simulink model "DC_DC_source_based_matrix_switches1"  (R2023b)
settings: Solver=FixedStepAuto  StartTime=0.0  StopTime=10000  FixedStep=0.01  RelTol=1e-3
InitFcn:
  | %run('D:\Thesis\main.m')
  | %run('E:\Thesis\main.m')
values from neighbouring files (symbols this model uses):
  cell_cap_Ah = 2.2    [find_maximum_ovlp.m]    (also in main.m)
  dst_q_cls = zeros(50, 2)    [main.m]
  dst_trg_soc_av = zeros(50, 1)    [main.m]
  soc = soc_in    [balance_costF.m]    (also in find_maximum_ovlp.m = fix(rand (1, cell_count) * 100); log_clustering.m; main.m = [16   16  50  27  27  23  22  73  73]; plot_final.m)
  src_q_cls = zeros(50, 2)    [main.m]
  src_trg_soc_av = zeros(50, 1)    [main.m]
undefined symbols (not defined in the file or in its folder): Ion, Lithium
libraries: spsIdealSwitchLib x18, spsBatteryLib x10, spsControlledCurrentSourceLib x4, spsVoltageMeasurementLib x4, simulink x2, slpidlib x1, spspowerguiLib x1
(part 2 of 2)

== matlab function DC_DC_source_based_matrix_switches1/DC-DC converter3/MATLAB Function ==
  data: enable input; current_left output; direction input; voltage_left input; voltage_right input; current_right output; current_desired input
function [current_left, current_right] = current_controller(enable, direction, voltage_left, voltage_right, current_desired)    
    current_left = 0;
    current_right = 0;
if(enable)
    %% left side sink, right side source
    if(direction == 0) 
        % variables definition
        current_source = -1 * current_desired;
        voltage_sink = voltage_left;
        voltage_source = voltage_right;

        % input and output power must match
        power_source = current_source * voltage_source;
        power_sink = power_source;
        if(voltage_sink  ~= 0)
            current_sink =  -1 * (power_sink / voltage_sink);
        else
            current_sink = -1 * current_source;
        end
        % power delivery
        if(current_sink > 0)
            current_sink = current_sink * -1;
        end
        if(current_source < 0)
            current_source = current_source * -1;
        end
        current_left = current_sink;
        current_right = current_source;
    %% left side source, right side sink
    elseif(direction == 1)
        % variables definition
        current_source = 1 * current_desired;
        voltage_sink = voltage_right;
        voltage_source = voltage_left;

        % input and output power must match
        power_source = current_source * voltage_source;
        power_sink = power_source;
        if(voltage_sink  ~= 0)
            current_sink =  -1 * (power_sink / voltage_sink);
        else
            current_sink = -1 * current_source;
        end

        % power delivery
        current_left = current_source;
        current_right = current_sink;
    end

else
    current_left = 0;
    current_right = 0;
end
end

== matlab function DC_DC_source_based_matrix_switches1/mcu/demux n ==
  data: u input; s1 output boolean; s2 output boolean; s3 output boolean; s4 output boolean; s5 output boolean; s6 output boolean; s7 output boolean; s8 output boolean; s9 output boolean
function [s1, s2, s3, s4, s5, s6, s7, s8, s9] = demux(u)

    switch(u)
        case 1
            s1 = true; s2 = false; s3 = false; s4 = false; s5 = false; s6 = false; s7 = false; s8 = false; s9 = false;
        case 2      	
            s1 = false; s2 = true; s3 = false; s4 = false; s5 = false; s6 = false; s7 = false; s8 = false; s9 = false;
        case 3      	
            s1 = false; s2 = false; s3 = true; s4 = false; s5 = false; s6 = false; s7 = false; s8 = false; s9 = false;
        case 4      	
            s1 = false; s2 = false; s3 = false; s4 = true; s5 = false; s6 = false; s7 = false; s8 = false; s9 = false;
        case 5      	
            s1 = false; s2 = false; s3 = false; s4 = false; s5 = true; s6 = false; s7 = false; s8 = false; s9 = false;
        case 6      	
            s1 = false; s2 = false; s3 = false; s4 = false; s5 = false; s6 = true; s7 = false; s8 = false; s9 = false;
        case 7      
            s1 = false; s2 = false; s3 = false; s4 = false; s5 = false; s6 = false; s7 = true; s8 = false; s9 = false;
        case 8      	
            s1 = false; s2 = false; s3 = false; s4 = false; s5 = false; s6 = false; s7 = false; s8 = true; s9 = false;
        case 9      
            s1 = false; s2 = false; s3 = false; s4 = false; s5 = false; s6 = false; s7 = false; s8 = false; s9 = true;
        otherwise   	
            s1 = false; s2 = false; s3 = false; s4 = false; s5 = false; s6 = false; s7 = false; s8 = false; s9 = false;
    end
end

== matlab function DC_DC_source_based_matrix_switches1/mcu/demux p ==
  data: u input; s1 output boolean; s2 output boolean; s3 output boolean; s4 output boolean; s5 output boolean; s6 output boolean; s7 output boolean; s8 output boolean; s9 output boolean
function [s1, s2, s3, s4, s5, s6, s7, s8, s9] = demux(u)

    switch(u)
        case 1
            s1 = true; s2 = false; s3 = false; s4 = false; s5 = false; s6 = false; s7 = false; s8 = false; s9 = false;
        case 2      	
            s1 = false; s2 = true; s3 = false; s4 = false; s5 = false; s6 = false; s7 = false; s8 = false; s9 = false;
        case 3      	
            s1 = false; s2 = false; s3 = true; s4 = false; s5 = false; s6 = false; s7 = false; s8 = false; s9 = false;
        case 4      	
            s1 = false; s2 = false; s3 = false; s4 = true; s5 = false; s6 = false; s7 = false; s8 = false; s9 = false;
        case 5      	
            s1 = false; s2 = false; s3 = false; s4 = false; s5 = true; s6 = false; s7 = false; s8 = false; s9 = false;
        case 6      	
            s1 = false; s2 = false; s3 = false; s4 = false; s5 = false; s6 = true; s7 = false; s8 = false; s9 = false;
        case 7      
            s1 = false; s2 = false; s3 = false; s4 = false; s5 = false; s6 = false; s7 = true; s8 = false; s9 = false;
        case 8      	
            s1 = false; s2 = false; s3 = false; s4 = false; s5 = false; s6 = false; s7 = false; s8 = true; s9 = false;
        case 9      
            s1 = false; s2 = false; s3 = false; s4 = false; s5 = false; s6 = false; s7 = false; s8 = false; s9 = true;
        otherwise   	
            s1 = false; s2 = false; s3 = false; s4 = false; s5 = false; s6 = false; s7 = false; s8 = false; s9 = false;
    end
end

== matlab function DC_DC_source_based_matrix_switches1/measurement/DC-DC converter/MATLAB Function ==
  data: enable input; current_left output; direction input; voltage_left input; voltage_right input; current_right output; current_desired input
function [current_left, current_right] = current_controller(enable, direction, voltage_left, voltage_right, current_desired)    
    current_left = 0;
    current_right = 0;
if(enable)
    %% left side sink, right side source
    if(direction == 0) 
        % variables definition
        current_sink = -1 * current_desired;
        voltage_sink = voltage_left;
        voltage_source = voltage_right;
        power_source = 0;
        power_sink = 0;

        % input and output power must match
        power_sink = current_sink * voltage_sink;
        power_source = power_sink;
        if(voltage_source ~= 0)
            current_source =  -1 * (power_source / voltage_source);
        else
            current_source = -1 * current_sink;
        end
        % power delivery
        if(current_sink > 0)
            current_sink = current_sink * -1;
        end
        if(current_source < 0)
            current_source = current_source * -1;
        end
        current_left = current_sink;
        current_right = current_source;
    %% left side source, right side sink
    elseif(direction == 1)
        % variables definition
        current_sink = -1 * current_desired;
        voltage_sink = voltage_right;
        voltage_source = voltage_left;
        power_source = 0;
        power_sink = 0;

        % input and output power must match
        power_sink = current_sink * voltage_sink;
        power_source = power_sink;
        if(voltage_source ~= 0)
            current_source =  -1 * (power_source / voltage_source);
        else
            current_source = -1 * current_sink;
        end
        % power delivery
        current_left = current_source;
        current_right = current_sink;
    end

else
    current_left = 0;
    current_right = 0;
end
end

== matlab function DC_DC_source_based_matrix_switches1/measurement/mcu/MATLAB Function ==
  data: destination_batts input; AH output; source_batts input; direction input
function AH = fcn(destination_batts, source_batts, direction)
AH_Base = 0.001;
AH = AH_Base;
source_batts_number = source_batts(1,2) - source_batts(1,1) + 1;
destination_batts_number = destination_batts(1,2) - destination_batts(1,1) + 1;


if source_batts_number > destination_batts_number && direction == 0 % draw less current from source 
    AH = destination_batts_number / source_batts_number * AH_Base;
elseif source_batts_number < destination_batts_number && direction == 1 % inject less current to destination
    AH = source_batts_number / destination_batts_number * AH_Base;
else 
    AH = AH_Base;
end
